simulink library "NxtrIMC"  (R2013b)
settings: Solver=ode45  StartTime=0.0  StopTime=10.0  RelTol=1e-3
settings Model: Creator=qzwc4r  LastModifiedBy=dz1yrm

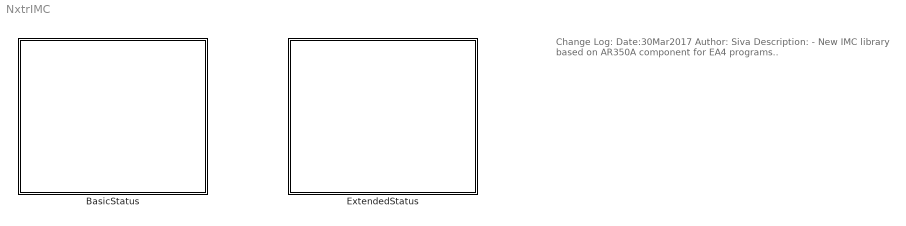
== system NxtrIMC ==
  note: Change Log:
      |
      | Date:30Mar2017
      | Author: Siva
      | Description:
      |      -  New IMC library based on AR350A component for EA4 programs..
  BasicStatus : Subsystem  TreatAsAtomicUnit=on
  ExtendedStatus : Subsystem  TreatAsAtomicUnit=on

== system NxtrIMC/BasicStatus ==
  note: To be used if Data signal is of datatype 'float32'
  note: To be used if Data signal is of datatype 'uint32'
  note: To be used if Data signal is of datatype 'int32'
  note: To be used if Data signal is of datatype 'uint16'
  note: To be used if Data signal is of datatype 'int16'
  note: To be used if Data signal is of datatype 'uint8'
  note: To be used if Data signal is of datatype 'int8'
  note: To be used if Data signal is of datatype 'boolean'
  GetSigImcDataf32 : Subsystem  mask(GetSigImcData_f32){DataVal=DataVal, StsVal=StsVal, RtnVal=RtnVal}
      mask prompts: DataVal "Data"; StsVal "Sts"; RtnVal "Return"
      mask help: Used to make a client call to IMC Arbitration function with basic status for float32 signals.
      mask init:
      | blk = gcb;
      | set_param([blk '/DataBlk'],'DataStoreName',DataVal)
      | set_param([blk '/StsBlk'],'DataStoreName',StsVal)
      | set_param([blk '/RtnBlk'],'DataStoreName',RtnVal)
      settings: AttributesFormatString=GetSigImcData_f32
  GetSigImcDatalogl : Subsystem  mask(GetSigImcData_logl){DataVal=DataVal, StsVal=StsVal, RtnVal=RtnVal}
      mask prompts: DataVal "Data"; StsVal "Sts"; RtnVal "Return"
      mask help: Used to make a client call to IMC Arbitration function with basic status for boolean signals.
      mask init:
      | blk = gcb;
      | set_param([blk '/DataBlk'],'DataStoreName',DataVal)
      | set_param([blk '/StsBlk'],'DataStoreName',StsVal)
      | set_param([blk '/RtnBlk'],'DataStoreName',RtnVal)
      settings: AttributesFormatString=GetSigImcData_logl
  GetSigImcDatas08 : Subsystem  mask(GetSigImcData_s08){DataVal=DataVal, StsVal=StsVal, RtnVal=RtnVal}
      mask prompts: DataVal "Data"; StsVal "Sts"; RtnVal "Return"
      mask help: Used to make a client call to IMC Arbitration function with basic status for int8 signals.
      mask init:
      | blk = gcb;
      | set_param([blk '/DataBlk'],'DataStoreName',DataVal)
      | set_param([blk '/StsBlk'],'DataStoreName',StsVal)
      | set_param([blk '/RtnBlk'],'DataStoreName',RtnVal)
      settings: AttributesFormatString=GetSigImcData_s08
  GetSigImcDatas16 : Subsystem  mask(GetSigImcData_s16){DataVal=DataVal, StsVal=StsVal, RtnVal=RtnVal}
      mask prompts: DataVal "Data"; StsVal "Sts"; RtnVal "Return"
      mask help: Used to make a client call to IMC Arbitration function with basic status for int16 signals.
      mask init:
      | blk = gcb;
      | set_param([blk '/DataBlk'],'DataStoreName',DataVal)
      | set_param([blk '/StsBlk'],'DataStoreName',StsVal)
      | set_param([blk '/RtnBlk'],'DataStoreName',RtnVal)
      settings: AttributesFormatString=GetSigImcData_s16
  GetSigImcDatas32 : Subsystem  mask(GetSigImcData_s32){DataVal=DataVal, StsVal=StsVal, RtnVal=RtnVal}
      mask prompts: DataVal "Data"; StsVal "Sts"; RtnVal "Return"
      mask help: Used to make a client call to IMC Arbitration function with basic status for int32 signals.
      mask init:
      | blk = gcb;
      | set_param([blk '/DataBlk'],'DataStoreName',DataVal)
      | set_param([blk '/StsBlk'],'DataStoreName',StsVal)
      | set_param([blk '/RtnBlk'],'DataStoreName',RtnVal)
      settings: AttributesFormatString=GetSigImcData_s32
  GetSigImcDatau08 : Subsystem  mask(GetSigImcData_u08){DataVal=DataVal, StsVal=StsVal, RtnVal=RtnVal}
      mask prompts: DataVal "Data"; StsVal "Sts"; RtnVal "Return"
      mask help: Used to make a client call to IMC Arbitration function with basic status for uint08 signals.
      mask init:
      | blk = gcb;
      | set_param([blk '/DataBlk'],'DataStoreName',DataVal)
      | set_param([blk '/StsBlk'],'DataStoreName',StsVal)
      | set_param([blk '/RtnBlk'],'DataStoreName',RtnVal)
      settings: AttributesFormatString=GetSigImcData_u08
  GetSigImcDatau16 : Subsystem  mask(GetSigImcData_u16){DataVal=DataVal, StsVal=StsVal, RtnVal=RtnVal}
      mask prompts: DataVal "Data"; StsVal "Sts"; RtnVal "Return"
      mask help: Used to make a client call to IMC Arbitration function with basic status for uint16 signals.
      mask init:
      | blk = gcb;
      | set_param([blk '/DataBlk'],'DataStoreName',DataVal)
      | set_param([blk '/StsBlk'],'DataStoreName',StsVal)
      | set_param([blk '/RtnBlk'],'DataStoreName',RtnVal)
      settings: AttributesFormatString=GetSigImcData_u16
  GetSigImcDatau32 : Subsystem  mask(GetSigImcData_u32){DataVal=DataVal, StsVal=StsVal, RtnVal=RtnVal}
      mask prompts: DataVal "Data"; StsVal "Sts"; RtnVal "Return"
      mask help: Used to make a client call to IMC Arbitration function with basic status for uint32 signals.
      mask init:
      | blk = gcb;
      | set_param([blk '/DataBlk'],'DataStoreName',DataVal)
      | set_param([blk '/StsBlk'],'DataStoreName',StsVal)
      | set_param([blk '/RtnBlk'],'DataStoreName',RtnVal)
      settings: AttributesFormatString=GetSigImcData_u32

== system NxtrIMC/ExtendedStatus ==
  note: To be used if Data signal is of datatype 'boolean'
  note: To be used if Data signal is of datatype 'int8'
  note: To be used if Data signal is of datatype 'uint8'
  note: To be used if Data signal is of datatype 'int16'
  note: To be used if Data signal is of datatype 'uint16'
  note: To be used if Data signal is of datatype 'int32'
  note: To be used if Data signal is of datatype 'uint32'
  note: To be used if Data signal is of datatype 'float32'
  GetSigImcDataf32 : Subsystem  mask(GetSigImcDataExtdSts_f32){DataVal=DataVal, StsVal=StsVal, DataSrcVal=DataSrcVal, RtnVal=RtnVal}
      mask prompts: DataVal "Data"; StsVal "Sts"; DataSrcVal "DataSrc"; RtnVal "Return"
      mask help: Used to make a client call to IMC Arbitration function with extended status for Float32 signals.
      mask init:
      | blk = gcb;
      | set_param([blk '/DataBlk'],'DataStoreName',DataVal)
      | set_param([blk '/StsBlk'],'DataStoreName',StsVal)
      | set_param([blk '/DataSrcBlk'],'DataStoreName',DataSrcVal)
      | set_param([blk '/RtnBlk'],'DataStoreName',RtnVal)
      settings: AttributesFormatString=GetSigImcDataExtdSts_f32
  GetSigImcDatalogl : Subsystem  mask(GetSigImcDataExtdSts_logl){DataVal=DataVal, StsVal=StsVal, DataSrcVal=DataSrcVal, RtnVal=RtnVal}
      mask prompts: DataVal "Data"; StsVal "Sts"; DataSrcVal "DataSrc"; RtnVal "Return"
      mask help: Used to make a client call to IMC Arbitration function with extended status for boolean signals.
      mask init: same as NxtrIMC/ExtendedStatus/GetSigImcDataf32
      settings: AttributesFormatString=GetSigImcDataExtdSts_logl
  GetSigImcDatas08 : Subsystem  mask(GetSigImcDataExtdSts_s08){DataVal=DataVal, StsVal=StsVal, DataSrcVal=DataSrcVal, RtnVal=RtnVal}
      mask prompts: DataVal "Data"; StsVal "Sts"; DataSrcVal "DataSrc"; RtnVal "Return"
      mask help: Used to make a client call to IMC Arbitration function with extended status for int8 signals.
      mask init: same as NxtrIMC/ExtendedStatus/GetSigImcDataf32
      settings: AttributesFormatString=GetSigImcDataExtdSts_s08
  GetSigImcDatas16 : Subsystem  mask(GetSigImcDataExtdSts_s16){DataVal=DataVal, StsVal=StsVal, DataSrcVal=DataSrcVal, RtnVal=RtnVal}
      mask prompts: DataVal "Data"; StsVal "Sts"; DataSrcVal "DataSrc"; RtnVal "Return"
      mask help: Used to make a client call to IMC Arbitration function with extended status for int16 signals.
      mask init: same as NxtrIMC/ExtendedStatus/GetSigImcDataf32
      settings: AttributesFormatString=GetSigImcDataExtdSts_s16
  GetSigImcDatas32 : Subsystem  mask(GetSigImcDataExtdSts_s32){DataVal=DataVal, StsVal=StsVal, DataSrcVal=DataSrcVal, RtnVal=RtnVal}
      mask prompts: DataVal "Data"; StsVal "Sts"; DataSrcVal "DataSrc"; RtnVal "Return"
      mask help: Used to make a client call to IMC Arbitration function with extended status for int32 signals.
      mask init: same as NxtrIMC/ExtendedStatus/GetSigImcDataf32
      settings: AttributesFormatString=GetSigImcDataExtdSts_s32
  GetSigImcDatau08 : Subsystem  mask(GetSigImcDataExtdSts_u08){DataVal=DataVal, StsVal=StsVal, DataSrcVal=DataSrcVal, RtnVal=RtnVal}
      mask prompts: DataVal "Data"; StsVal "Sts"; DataSrcVal "DataSrc"; RtnVal "Return"
      mask help: Used to make a client call to IMC Arbitration function with extended status for uint8 signals.
      mask init: same as NxtrIMC/ExtendedStatus/GetSigImcDataf32
      settings: AttributesFormatString=GetSigImcDataExtdSts_u08
  GetSigImcDatau16 : Subsystem  mask(GetSigImcDataExtdSts_u16){DataVal=DataVal, StsVal=StsVal, DataSrcVal=DataSrcVal, RtnVal=RtnVal}
      mask prompts: DataVal "Data"; StsVal "Sts"; DataSrcVal "DataSrc"; RtnVal "Return"
      mask help: Used to make a client call to IMC Arbitration function with extended status for uint16 signals.
      mask init: same as NxtrIMC/ExtendedStatus/GetSigImcDataf32
      settings: AttributesFormatString=GetSigImcDataExtdSts_u16
  GetSigImcDatau32 : Subsystem  mask(GetSigImcDataExtdSts_u32){DataVal=DataVal, StsVal=StsVal, DataSrcVal=DataSrcVal, RtnVal=RtnVal}
      mask prompts: DataVal "Data"; StsVal "Sts"; DataSrcVal "DataSrc"; RtnVal "Return"
      mask help: Used to make a client call to IMC Arbitration function with extended status for uint32 signals.
      mask init: same as NxtrIMC/ExtendedStatus/GetSigImcDataf32
      settings: AttributesFormatString=GetSigImcDataExtdSts_u32

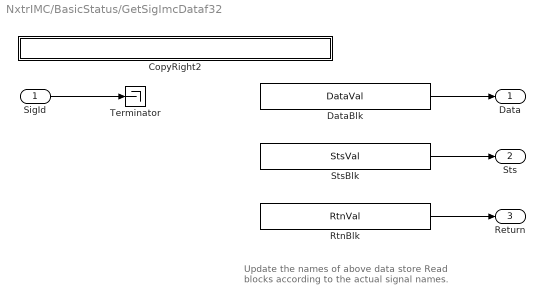
== system NxtrIMC/BasicStatus/GetSigImcDataf32 ==
  note: Update the names of above data store Read
      | blocks according to the actual signal names.
  SigId : Inport
  CopyRight2 : Subsystem  Description=|  mask(Copyright Information){none=on}
      | Copyright info block.                                               
      |                                                                     
      | Place copyright information at the top of every subsystem in design.
      mask prompts: none "No parameters"
      mask help: Place copyright information at the top of every subsystem in design.
      mask Display:
      | NxtrConf = 'Nexteer Confidential';
      | 
      | sys = bdroot; %handle for the current model ("system")
      | first = get_param(sys,'Created');
      | first = first(end-3:end);  %year is last four digits
      | 
      | last = get_param(sys,'LastModifiedDate');
      | if isempty(last)
      |     last = datestr(now,'yyyy');
      | else
      |     last = last(end-3:end);
      | end
      | 
      | if strcmp(first,last)
      |     fprintf('%s -- Copyright %s Nexteer',NxtrConf,first)
      | else
      |     fprintf('%s -- %s%s- %s Nexteer',NxtrConf,char(169),first,last)
      | end
  DataBlk : DataStoreRead  DataStoreName=DataVal
  RtnBlk : DataStoreRead  DataStoreName=RtnVal
  StsBlk : DataStoreRead  DataStoreName=StsVal
  Terminator : Terminator
  Data : Outport
  Sts : Outport  Port=2  OutDataTypeStr=Enum: ImcArbnRxSts1
  Return : Outport  Port=3
  wires:
  SigId/1 -> Terminator/1
  StsBlk/1 -> Sts/1
  DataBlk/1 -> Data/1
  RtnBlk/1 -> Return/1

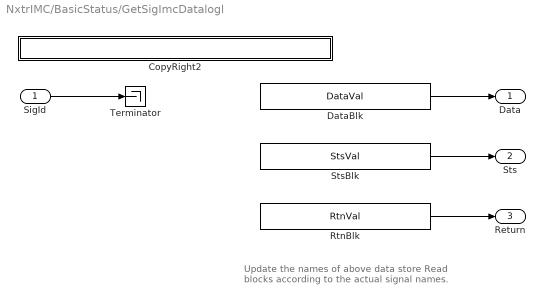
== system NxtrIMC/BasicStatus/GetSigImcDatalogl ==
  note: Update the names of above data store Read
      | blocks according to the actual signal names.
  SigId : Inport
  CopyRight2 : Subsystem  Description=|  mask(Copyright Information){none=on}
      | Copyright info block.                                               
      |                                                                     
      | Place copyright information at the top of every subsystem in design.
      mask prompts: none "No parameters"
      mask help: Place copyright information at the top of every subsystem in design.
      mask Display:
      | NxtrConf = 'Nexteer Confidential';
      | 
      | sys = bdroot; %handle for the current model ("system")
      | first = get_param(sys,'Created');
      | first = first(end-3:end);  %year is last four digits
      | 
      | last = get_param(sys,'LastModifiedDate');
      | if isempty(last)
      |     last = datestr(now,'yyyy');
      | else
      |     last = last(end-3:end);
      | end
      | 
      | if strcmp(first,last)
      |     fprintf('%s -- Copyright %s Nexteer',NxtrConf,first)
      | else
      |     fprintf('%s -- %s%s- %s Nexteer',NxtrConf,char(169),first,last)
      | end
  DataBlk : DataStoreRead  DataStoreName=DataVal
  RtnBlk : DataStoreRead  DataStoreName=RtnVal
  StsBlk : DataStoreRead  DataStoreName=StsVal
  Terminator : Terminator
  Data : Outport
  Sts : Outport  Port=2  OutDataTypeStr=Enum: ImcArbnRxSts1
  Return : Outport  Port=3
  wires:
  SigId/1 -> Terminator/1
  StsBlk/1 -> Sts/1
  DataBlk/1 -> Data/1
  RtnBlk/1 -> Return/1

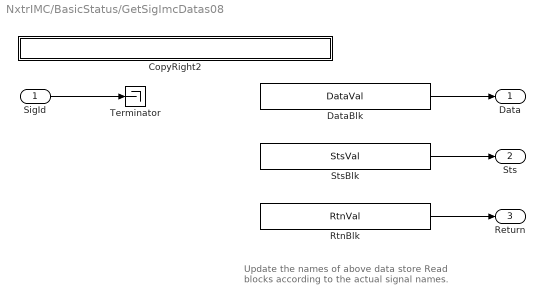
== system NxtrIMC/BasicStatus/GetSigImcDatas08 ==
  note: Update the names of above data store Read
      | blocks according to the actual signal names.
  SigId : Inport
  CopyRight2 : Subsystem  Description=|  mask(Copyright Information){none=on}
      | Copyright info block.                                               
      |                                                                     
      | Place copyright information at the top of every subsystem in design.
      mask prompts: none "No parameters"
      mask help: Place copyright information at the top of every subsystem in design.
      mask Display:
      | NxtrConf = 'Nexteer Confidential';
      | 
      | sys = bdroot; %handle for the current model ("system")
      | first = get_param(sys,'Created');
      | first = first(end-3:end);  %year is last four digits
      | 
      | last = get_param(sys,'LastModifiedDate');
      | if isempty(last)
      |     last = datestr(now,'yyyy');
      | else
      |     last = last(end-3:end);
      | end
      | 
      | if strcmp(first,last)
      |     fprintf('%s -- Copyright %s Nexteer',NxtrConf,first)
      | else
      |     fprintf('%s -- %s%s- %s Nexteer',NxtrConf,char(169),first,last)
      | end
  DataBlk : DataStoreRead  DataStoreName=DataVal
  RtnBlk : DataStoreRead  DataStoreName=RtnVal
  StsBlk : DataStoreRead  DataStoreName=StsVal
  Terminator : Terminator
  Data : Outport
  Sts : Outport  Port=2  OutDataTypeStr=Enum: ImcArbnRxSts1
  Return : Outport  Port=3
  wires:
  SigId/1 -> Terminator/1
  StsBlk/1 -> Sts/1
  DataBlk/1 -> Data/1
  RtnBlk/1 -> Return/1

== system NxtrIMC/BasicStatus/GetSigImcDatas16 ==
  note: Update the names of above data store Read
      | blocks according to the actual signal names.
  SigId : Inport
  CopyRight2 : Subsystem  Description=|  mask(Copyright Information){none=on}
      | Copyright info block.                                               
      |                                                                     
      | Place copyright information at the top of every subsystem in design.
      mask prompts: none "No parameters"
      mask help: Place copyright information at the top of every subsystem in design.
      mask Display:
      | NxtrConf = 'Nexteer Confidential';
      | 
      | sys = bdroot; %handle for the current model ("system")
      | first = get_param(sys,'Created');
      | first = first(end-3:end);  %year is last four digits
      | 
      | last = get_param(sys,'LastModifiedDate');
      | if isempty(last)
      |     last = datestr(now,'yyyy');
      | else
      |     last = last(end-3:end);
      | end
      | 
      | if strcmp(first,last)
      |     fprintf('%s -- Copyright %s Nexteer',NxtrConf,first)
      | else
      |     fprintf('%s -- %s%s- %s Nexteer',NxtrConf,char(169),first,last)
      | end
  DataBlk : DataStoreRead  DataStoreName=DataVal
  RtnBlk : DataStoreRead  DataStoreName=RtnVal
  StsBlk : DataStoreRead  DataStoreName=StsVal
  Terminator : Terminator
  Data : Outport
  Sts : Outport  Port=2  OutDataTypeStr=Enum: ImcArbnRxSts1
  Return : Outport  Port=3
  wires:
  SigId/1 -> Terminator/1
  StsBlk/1 -> Sts/1
  DataBlk/1 -> Data/1
  RtnBlk/1 -> Return/1

== system NxtrIMC/BasicStatus/GetSigImcDatas32 ==
  note: Update the names of above data store Read
      | blocks according to the actual signal names.
  SigId : Inport
  CopyRight2 : Subsystem  Description=|  mask(Copyright Information){none=on}
      | Copyright info block.                                               
      |                                                                     
      | Place copyright information at the top of every subsystem in design.
      mask prompts: none "No parameters"
      mask help: Place copyright information at the top of every subsystem in design.
      mask Display:
      | NxtrConf = 'Nexteer Confidential';
      | 
      | sys = bdroot; %handle for the current model ("system")
      | first = get_param(sys,'Created');
      | first = first(end-3:end);  %year is last four digits
      | 
      | last = get_param(sys,'LastModifiedDate');
      | if isempty(last)
      |     last = datestr(now,'yyyy');
      | else
      |     last = last(end-3:end);
      | end
      | 
      | if strcmp(first,last)
      |     fprintf('%s -- Copyright %s Nexteer',NxtrConf,first)
      | else
      |     fprintf('%s -- %s%s- %s Nexteer',NxtrConf,char(169),first,last)
      | end
  DataBlk : DataStoreRead  DataStoreName=DataVal
  RtnBlk : DataStoreRead  DataStoreName=RtnVal
  StsBlk : DataStoreRead  DataStoreName=StsVal
  Terminator : Terminator
  Data : Outport
  Sts : Outport  Port=2  OutDataTypeStr=Enum: ImcArbnRxSts1
  Return : Outport  Port=3
  wires:
  SigId/1 -> Terminator/1
  StsBlk/1 -> Sts/1
  DataBlk/1 -> Data/1
  RtnBlk/1 -> Return/1

== system NxtrIMC/BasicStatus/GetSigImcDatau08 ==
  note: Update the names of above data store Read
      | blocks according to the actual signal names.
  SigId : Inport
  CopyRight2 : Subsystem  Description=|  mask(Copyright Information){none=on}
      | Copyright info block.                                               
      |                                                                     
      | Place copyright information at the top of every subsystem in design.
      mask prompts: none "No parameters"
      mask help: Place copyright information at the top of every subsystem in design.
      mask Display:
      | NxtrConf = 'Nexteer Confidential';
      | 
      | sys = bdroot; %handle for the current model ("system")
      | first = get_param(sys,'Created');
      | first = first(end-3:end);  %year is last four digits
      | 
      | last = get_param(sys,'LastModifiedDate');
      | if isempty(last)
      |     last = datestr(now,'yyyy');
      | else
      |     last = last(end-3:end);
      | end
      | 
      | if strcmp(first,last)
      |     fprintf('%s -- Copyright %s Nexteer',NxtrConf,first)
      | else
      |     fprintf('%s -- %s%s- %s Nexteer',NxtrConf,char(169),first,last)
      | end
  DataBlk : DataStoreRead  DataStoreName=DataVal
  RtnBlk : DataStoreRead  DataStoreName=RtnVal
  StsBlk : DataStoreRead  DataStoreName=StsVal
  Terminator : Terminator
  Data : Outport
  Sts : Outport  Port=2  OutDataTypeStr=Enum: ImcArbnRxSts1
  Return : Outport  Port=3
  wires:
  SigId/1 -> Terminator/1
  StsBlk/1 -> Sts/1
  DataBlk/1 -> Data/1
  RtnBlk/1 -> Return/1

== system NxtrIMC/BasicStatus/GetSigImcDatau16 ==
  note: Update the names of above data store Read
      | blocks according to the actual signal names.
  SigId : Inport
  CopyRight2 : Subsystem  Description=|  mask(Copyright Information){none=on}
      | Copyright info block.                                               
      |                                                                     
      | Place copyright information at the top of every subsystem in design.
      mask prompts: none "No parameters"
      mask help: Place copyright information at the top of every subsystem in design.
      mask Display:
      | NxtrConf = 'Nexteer Confidential';
      | 
      | sys = bdroot; %handle for the current model ("system")
      | first = get_param(sys,'Created');
      | first = first(end-3:end);  %year is last four digits
      | 
      | last = get_param(sys,'LastModifiedDate');
      | if isempty(last)
      |     last = datestr(now,'yyyy');
      | else
      |     last = last(end-3:end);
      | end
      | 
      | if strcmp(first,last)
      |     fprintf('%s -- Copyright %s Nexteer',NxtrConf,first)
      | else
      |     fprintf('%s -- %s%s- %s Nexteer',NxtrConf,char(169),first,last)
      | end
  DataBlk : DataStoreRead  DataStoreName=DataVal
  RtnBlk : DataStoreRead  DataStoreName=RtnVal
  StsBlk : DataStoreRead  DataStoreName=StsVal
  Terminator : Terminator
  Data : Outport
  Sts : Outport  Port=2  OutDataTypeStr=Enum: ImcArbnRxSts1
  Return : Outport  Port=3
  wires:
  SigId/1 -> Terminator/1
  StsBlk/1 -> Sts/1
  DataBlk/1 -> Data/1
  RtnBlk/1 -> Return/1

== system NxtrIMC/BasicStatus/GetSigImcDatau32 ==
  note: Update the names of above data store Read
      | blocks according to the actual signal names.
  SigId : Inport
  CopyRight2 : Subsystem  Description=|  mask(Copyright Information){none=on}
      | Copyright info block.                                               
      |                                                                     
      | Place copyright information at the top of every subsystem in design.
      mask prompts: none "No parameters"
      mask help: Place copyright information at the top of every subsystem in design.
      mask Display:
      | NxtrConf = 'Nexteer Confidential';
      | 
      | sys = bdroot; %handle for the current model ("system")
      | first = get_param(sys,'Created');
      | first = first(end-3:end);  %year is last four digits
      | 
      | last = get_param(sys,'LastModifiedDate');
      | if isempty(last)
      |     last = datestr(now,'yyyy');
      | else
      |     last = last(end-3:end);
      | end
      | 
      | if strcmp(first,last)
      |     fprintf('%s -- Copyright %s Nexteer',NxtrConf,first)
      | else
      |     fprintf('%s -- %s%s- %s Nexteer',NxtrConf,char(169),first,last)
      | end
  DataBlk : DataStoreRead  DataStoreName=DataVal
  RtnBlk : DataStoreRead  DataStoreName=RtnVal
  StsBlk : DataStoreRead  DataStoreName=StsVal
  Terminator : Terminator
  Data : Outport
  Sts : Outport  Port=2  OutDataTypeStr=Enum: ImcArbnRxSts1
  Return : Outport  Port=3
  wires:
  SigId/1 -> Terminator/1
  StsBlk/1 -> Sts/1
  DataBlk/1 -> Data/1
  RtnBlk/1 -> Return/1

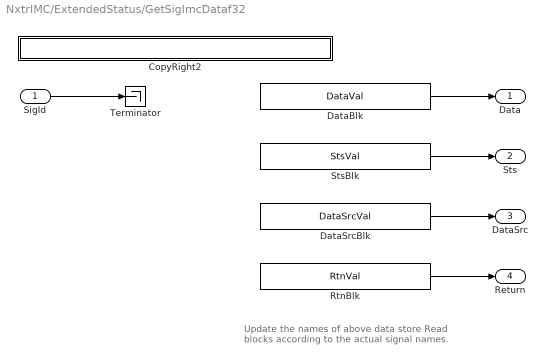
== system NxtrIMC/ExtendedStatus/GetSigImcDataf32 ==
  note: Update the names of above data store Read
      | blocks according to the actual signal names.
  SigId : Inport
  CopyRight2 : Subsystem  Description=|  mask(Copyright Information){none=on}
      | Copyright info block.                                               
      |                                                                     
      | Place copyright information at the top of every subsystem in design.
      mask prompts: none "No parameters"
      mask help: Place copyright information at the top of every subsystem in design.
      mask Display:
      | NxtrConf = 'Nexteer Confidential';
      | 
      | sys = bdroot; %handle for the current model ("system")
      | first = get_param(sys,'Created');
      | first = first(end-3:end);  %year is last four digits
      | 
      | last = get_param(sys,'LastModifiedDate');
      | if isempty(last)
      |     last = datestr(now,'yyyy');
      | else
      |     last = last(end-3:end);
      | end
      | 
      | if strcmp(first,last)
      |     fprintf('%s -- Copyright %s Nexteer',NxtrConf,first)
      | else
      |     fprintf('%s -- %s%s- %s Nexteer',NxtrConf,char(169),first,last)
      | end
  DataBlk : DataStoreRead  DataStoreName=DataVal
  DataSrcBlk : DataStoreRead  DataStoreName=DataSrcVal
  RtnBlk : DataStoreRead  DataStoreName=RtnVal
  StsBlk : DataStoreRead  DataStoreName=StsVal
  Terminator : Terminator
  Data : Outport
  Sts : Outport  Port=2  OutDataTypeStr=Enum: ImcArbnRxExtdSts1
  DataSrc : Outport  Port=3  OutDataTypeStr=Enum: ImcArbnRxDataSrc1
  Return : Outport  Port=4
  wires:
  SigId/1 -> Terminator/1
  StsBlk/1 -> Sts/1
  DataBlk/1 -> Data/1
  RtnBlk/1 -> Return/1
  DataSrcBlk/1 -> DataSrc/1

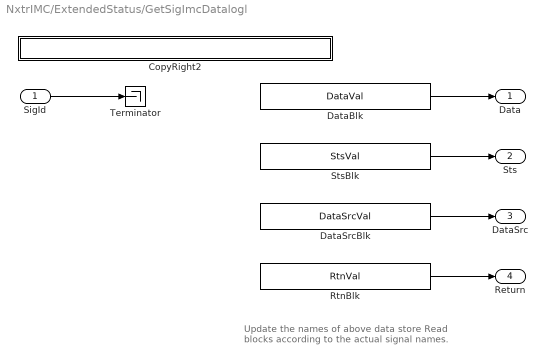
== system NxtrIMC/ExtendedStatus/GetSigImcDatalogl ==
  note: Update the names of above data store Read
      | blocks according to the actual signal names.
  SigId : Inport
  CopyRight2 : Subsystem  Description=|  mask(Copyright Information){none=on}
      | Copyright info block.                                               
      |                                                                     
      | Place copyright information at the top of every subsystem in design.
      mask prompts: none "No parameters"
      mask help: Place copyright information at the top of every subsystem in design.
      mask Display:
      | NxtrConf = 'Nexteer Confidential';
      | 
      | sys = bdroot; %handle for the current model ("system")
      | first = get_param(sys,'Created');
      | first = first(end-3:end);  %year is last four digits
      | 
      | last = get_param(sys,'LastModifiedDate');
      | if isempty(last)
      |     last = datestr(now,'yyyy');
      | else
      |     last = last(end-3:end);
      | end
      | 
      | if strcmp(first,last)
      |     fprintf('%s -- Copyright %s Nexteer',NxtrConf,first)
      | else
      |     fprintf('%s -- %s%s- %s Nexteer',NxtrConf,char(169),first,last)
      | end
  DataBlk : DataStoreRead  DataStoreName=DataVal
  DataSrcBlk : DataStoreRead  DataStoreName=DataSrcVal
  RtnBlk : DataStoreRead  DataStoreName=RtnVal
  StsBlk : DataStoreRead  DataStoreName=StsVal
  Terminator : Terminator
  Data : Outport
  Sts : Outport  Port=2  OutDataTypeStr=Enum: ImcArbnRxExtdSts1
  DataSrc : Outport  Port=3  OutDataTypeStr=Enum: ImcArbnRxDataSrc1
  Return : Outport  Port=4
  wires:
  SigId/1 -> Terminator/1
  StsBlk/1 -> Sts/1
  DataBlk/1 -> Data/1
  RtnBlk/1 -> Return/1
  DataSrcBlk/1 -> DataSrc/1

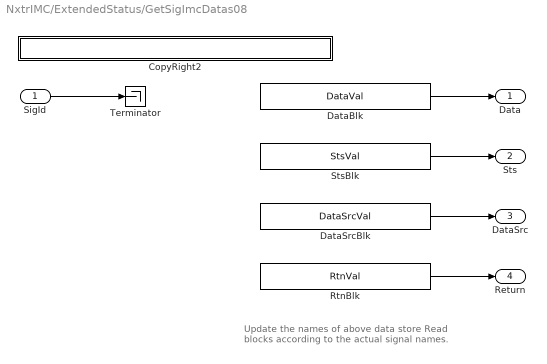
== system NxtrIMC/ExtendedStatus/GetSigImcDatas08 ==
  note: Update the names of above data store Read
      | blocks according to the actual signal names.
  SigId : Inport
  CopyRight2 : Subsystem  Description=|  mask(Copyright Information){none=on}
      | Copyright info block.                                               
      |                                                                     
      | Place copyright information at the top of every subsystem in design.
      mask prompts: none "No parameters"
      mask help: Place copyright information at the top of every subsystem in design.
      mask Display:
      | NxtrConf = 'Nexteer Confidential';
      | 
      | sys = bdroot; %handle for the current model ("system")
      | first = get_param(sys,'Created');
      | first = first(end-3:end);  %year is last four digits
      | 
      | last = get_param(sys,'LastModifiedDate');
      | if isempty(last)
      |     last = datestr(now,'yyyy');
      | else
      |     last = last(end-3:end);
      | end
      | 
      | if strcmp(first,last)
      |     fprintf('%s -- Copyright %s Nexteer',NxtrConf,first)
      | else
      |     fprintf('%s -- %s%s- %s Nexteer',NxtrConf,char(169),first,last)
      | end
  DataBlk : DataStoreRead  DataStoreName=DataVal
  DataSrcBlk : DataStoreRead  DataStoreName=DataSrcVal
  RtnBlk : DataStoreRead  DataStoreName=RtnVal
  StsBlk : DataStoreRead  DataStoreName=StsVal
  Terminator : Terminator
  Data : Outport
  Sts : Outport  Port=2  OutDataTypeStr=Enum: ImcArbnRxExtdSts1
  DataSrc : Outport  Port=3  OutDataTypeStr=Enum: ImcArbnRxDataSrc1
  Return : Outport  Port=4
  wires:
  SigId/1 -> Terminator/1
  StsBlk/1 -> Sts/1
  DataBlk/1 -> Data/1
  RtnBlk/1 -> Return/1
  DataSrcBlk/1 -> DataSrc/1

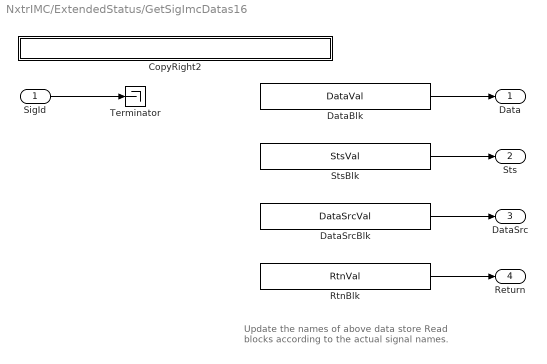
== system NxtrIMC/ExtendedStatus/GetSigImcDatas16 ==
  note: Update the names of above data store Read
      | blocks according to the actual signal names.
  SigId : Inport
  CopyRight2 : Subsystem  Description=|  mask(Copyright Information){none=on}
      | Copyright info block.                                               
      |                                                                     
      | Place copyright information at the top of every subsystem in design.
      mask prompts: none "No parameters"
      mask help: Place copyright information at the top of every subsystem in design.
      mask Display:
      | NxtrConf = 'Nexteer Confidential';
      | 
      | sys = bdroot; %handle for the current model ("system")
      | first = get_param(sys,'Created');
      | first = first(end-3:end);  %year is last four digits
      | 
      | last = get_param(sys,'LastModifiedDate');
      | if isempty(last)
      |     last = datestr(now,'yyyy');
      | else
      |     last = last(end-3:end);
      | end
      | 
      | if strcmp(first,last)
      |     fprintf('%s -- Copyright %s Nexteer',NxtrConf,first)
      | else
      |     fprintf('%s -- %s%s- %s Nexteer',NxtrConf,char(169),first,last)
      | end
  DataBlk : DataStoreRead  DataStoreName=DataVal
  DataSrcBlk : DataStoreRead  DataStoreName=DataSrcVal
  RtnBlk : DataStoreRead  DataStoreName=RtnVal
  StsBlk : DataStoreRead  DataStoreName=StsVal
  Terminator : Terminator
  Data : Outport
  Sts : Outport  Port=2  OutDataTypeStr=Enum: ImcArbnRxExtdSts1
  DataSrc : Outport  Port=3  OutDataTypeStr=Enum: ImcArbnRxDataSrc1
  Return : Outport  Port=4
  wires:
  SigId/1 -> Terminator/1
  StsBlk/1 -> Sts/1
  DataBlk/1 -> Data/1
  RtnBlk/1 -> Return/1
  DataSrcBlk/1 -> DataSrc/1

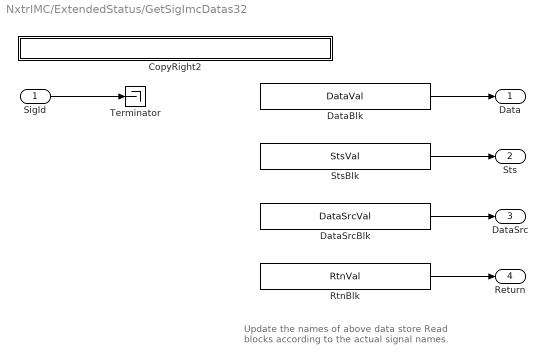
== system NxtrIMC/ExtendedStatus/GetSigImcDatas32 ==
  note: Update the names of above data store Read
      | blocks according to the actual signal names.
  SigId : Inport
  CopyRight2 : Subsystem  Description=|  mask(Copyright Information){none=on}
      | Copyright info block.                                               
      |                                                                     
      | Place copyright information at the top of every subsystem in design.
      mask prompts: none "No parameters"
      mask help: Place copyright information at the top of every subsystem in design.
      mask Display:
      | NxtrConf = 'Nexteer Confidential';
      | 
      | sys = bdroot; %handle for the current model ("system")
      | first = get_param(sys,'Created');
      | first = first(end-3:end);  %year is last four digits
      | 
      | last = get_param(sys,'LastModifiedDate');
      | if isempty(last)
      |     last = datestr(now,'yyyy');
      | else
      |     last = last(end-3:end);
      | end
      | 
      | if strcmp(first,last)
      |     fprintf('%s -- Copyright %s Nexteer',NxtrConf,first)
      | else
      |     fprintf('%s -- %s%s- %s Nexteer',NxtrConf,char(169),first,last)
      | end
  DataBlk : DataStoreRead  DataStoreName=DataVal
  DataSrcBlk : DataStoreRead  DataStoreName=DataSrcVal
  RtnBlk : DataStoreRead  DataStoreName=RtnVal
  StsBlk : DataStoreRead  DataStoreName=StsVal
  Terminator : Terminator
  Data : Outport
  Sts : Outport  Port=2  OutDataTypeStr=Enum: ImcArbnRxExtdSts1
  DataSrc : Outport  Port=3  OutDataTypeStr=Enum: ImcArbnRxDataSrc1
  Return : Outport  Port=4
  wires:
  SigId/1 -> Terminator/1
  StsBlk/1 -> Sts/1
  DataBlk/1 -> Data/1
  RtnBlk/1 -> Return/1
  DataSrcBlk/1 -> DataSrc/1

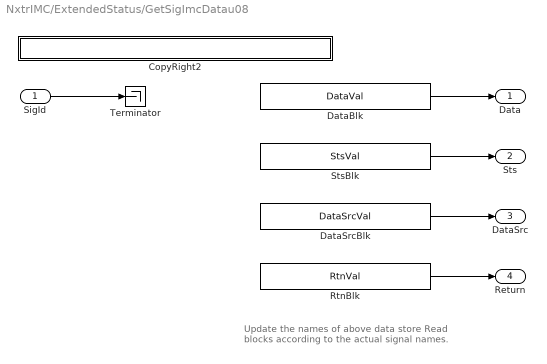
== system NxtrIMC/ExtendedStatus/GetSigImcDatau08 ==
  note: Update the names of above data store Read
      | blocks according to the actual signal names.
  SigId : Inport
  CopyRight2 : Subsystem  Description=|  mask(Copyright Information){none=on}
      | Copyright info block.                                               
      |                                                                     
      | Place copyright information at the top of every subsystem in design.
      mask prompts: none "No parameters"
      mask help: Place copyright information at the top of every subsystem in design.
      mask Display:
      | NxtrConf = 'Nexteer Confidential';
      | 
      | sys = bdroot; %handle for the current model ("system")
      | first = get_param(sys,'Created');
      | first = first(end-3:end);  %year is last four digits
      | 
      | last = get_param(sys,'LastModifiedDate');
      | if isempty(last)
      |     last = datestr(now,'yyyy');
      | else
      |     last = last(end-3:end);
      | end
      | 
      | if strcmp(first,last)
      |     fprintf('%s -- Copyright %s Nexteer',NxtrConf,first)
      | else
      |     fprintf('%s -- %s%s- %s Nexteer',NxtrConf,char(169),first,last)
      | end
  DataBlk : DataStoreRead  DataStoreName=DataVal
  DataSrcBlk : DataStoreRead  DataStoreName=DataSrcVal
  RtnBlk : DataStoreRead  DataStoreName=RtnVal
  StsBlk : DataStoreRead  DataStoreName=StsVal
  Terminator : Terminator
  Data : Outport
  Sts : Outport  Port=2  OutDataTypeStr=Enum: ImcArbnRxExtdSts1
  DataSrc : Outport  Port=3  OutDataTypeStr=Enum: ImcArbnRxDataSrc1
  Return : Outport  Port=4
  wires:
  SigId/1 -> Terminator/1
  StsBlk/1 -> Sts/1
  DataBlk/1 -> Data/1
  RtnBlk/1 -> Return/1
  DataSrcBlk/1 -> DataSrc/1

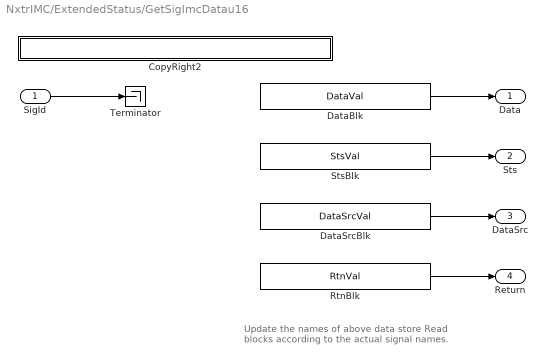
== system NxtrIMC/ExtendedStatus/GetSigImcDatau16 ==
  note: Update the names of above data store Read
      | blocks according to the actual signal names.
  SigId : Inport
  CopyRight2 : Subsystem  Description=|  mask(Copyright Information){none=on}
      | Copyright info block.                                               
      |                                                                     
      | Place copyright information at the top of every subsystem in design.
      mask prompts: none "No parameters"
      mask help: Place copyright information at the top of every subsystem in design.
      mask Display:
      | NxtrConf = 'Nexteer Confidential';
      | 
      | sys = bdroot; %handle for the current model ("system")
      | first = get_param(sys,'Created');
      | first = first(end-3:end);  %year is last four digits
      | 
      | last = get_param(sys,'LastModifiedDate');
      | if isempty(last)
      |     last = datestr(now,'yyyy');
      | else
      |     last = last(end-3:end);
      | end
      | 
      | if strcmp(first,last)
      |     fprintf('%s -- Copyright %s Nexteer',NxtrConf,first)
      | else
      |     fprintf('%s -- %s%s- %s Nexteer',NxtrConf,char(169),first,last)
      | end
  DataBlk : DataStoreRead  DataStoreName=DataVal
  DataSrcBlk : DataStoreRead  DataStoreName=DataSrcVal
  RtnBlk : DataStoreRead  DataStoreName=RtnVal
  StsBlk : DataStoreRead  DataStoreName=StsVal
  Terminator : Terminator
  Data : Outport
  Sts : Outport  Port=2  OutDataTypeStr=Enum: ImcArbnRxExtdSts1
  DataSrc : Outport  Port=3  OutDataTypeStr=Enum: ImcArbnRxDataSrc1
  Return : Outport  Port=4
  wires:
  SigId/1 -> Terminator/1
  StsBlk/1 -> Sts/1
  DataBlk/1 -> Data/1
  RtnBlk/1 -> Return/1
  DataSrcBlk/1 -> DataSrc/1

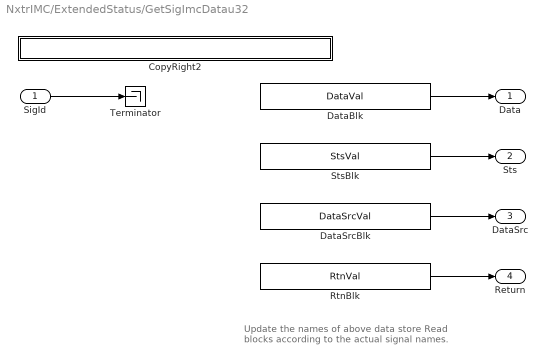
== system NxtrIMC/ExtendedStatus/GetSigImcDatau32 ==
  note: Update the names of above data store Read
      | blocks according to the actual signal names.
  SigId : Inport
  CopyRight2 : Subsystem  Description=|  mask(Copyright Information){none=on}
      | Copyright info block.                                               
      |                                                                     
      | Place copyright information at the top of every subsystem in design.
      mask prompts: none "No parameters"
      mask help: Place copyright information at the top of every subsystem in design.
      mask Display:
      | NxtrConf = 'Nexteer Confidential';
      | 
      | sys = bdroot; %handle for the current model ("system")
      | first = get_param(sys,'Created');
      | first = first(end-3:end);  %year is last four digits
      | 
      | last = get_param(sys,'LastModifiedDate');
      | if isempty(last)
      |     last = datestr(now,'yyyy');
      | else
      |     last = last(end-3:end);
      | end
      | 
      | if strcmp(first,last)
      |     fprintf('%s -- Copyright %s Nexteer',NxtrConf,first)
      | else
      |     fprintf('%s -- %s%s- %s Nexteer',NxtrConf,char(169),first,last)
      | end
  DataBlk : DataStoreRead  DataStoreName=DataVal
  DataSrcBlk : DataStoreRead  DataStoreName=DataSrcVal
  RtnBlk : DataStoreRead  DataStoreName=RtnVal
  StsBlk : DataStoreRead  DataStoreName=StsVal
  Terminator : Terminator
  Data : Outport
  Sts : Outport  Port=2  OutDataTypeStr=Enum: ImcArbnRxExtdSts1
  DataSrc : Outport  Port=3  OutDataTypeStr=Enum: ImcArbnRxDataSrc1
  Return : Outport  Port=4
  wires:
  SigId/1 -> Terminator/1
  StsBlk/1 -> Sts/1
  DataBlk/1 -> Data/1
  RtnBlk/1 -> Return/1
  DataSrcBlk/1 -> DataSrc/1

== system NxtrIMC/BasicStatus/GetSigImcDataf32/CopyRight2 ==

== system NxtrIMC/BasicStatus/GetSigImcDatalogl/CopyRight2 ==

== system NxtrIMC/BasicStatus/GetSigImcDatas08/CopyRight2 ==

== system NxtrIMC/BasicStatus/GetSigImcDatas16/CopyRight2 ==

== system NxtrIMC/BasicStatus/GetSigImcDatas32/CopyRight2 ==

== system NxtrIMC/BasicStatus/GetSigImcDatau08/CopyRight2 ==

== system NxtrIMC/BasicStatus/GetSigImcDatau16/CopyRight2 ==

== system NxtrIMC/BasicStatus/GetSigImcDatau32/CopyRight2 ==

== system NxtrIMC/ExtendedStatus/GetSigImcDataf32/CopyRight2 ==

== system NxtrIMC/ExtendedStatus/GetSigImcDatalogl/CopyRight2 ==

== system NxtrIMC/ExtendedStatus/GetSigImcDatas08/CopyRight2 ==

== system NxtrIMC/ExtendedStatus/GetSigImcDatas16/CopyRight2 ==

== system NxtrIMC/ExtendedStatus/GetSigImcDatas32/CopyRight2 ==

== system NxtrIMC/ExtendedStatus/GetSigImcDatau08/CopyRight2 ==

== system NxtrIMC/ExtendedStatus/GetSigImcDatau16/CopyRight2 ==

== system NxtrIMC/ExtendedStatus/GetSigImcDatau32/CopyRight2 ==
